simulink model "sg_xsvi_fanout"  (Simulink 7.6)
settings: Solver=ode45  StartTime=0.0  StopTime=1600.0  RelTol=1e-3
undefined symbols (not defined in the file): gcbh, xlBlockLoadCallback, xlGetNormalizedPeriod
libraries: xbsIndex_r4 x41, dspsrcs4 x6
settings Model: Creator=tbooth  LastModifiedBy=tawassne
settings OptimizationCC: InitFltsAndDblsToZero=on
settings DebuggingCC: SaveWithParameterizedLinksMsg=none  SignalResolutionControl=TryResolveAllWithWarning  MultiTaskDSMMsg=warning  MultiTaskCondExecSysMsg=none  StrictBusMsg=Warning
settings RTWCC: IncludeERTFirstTime=on
settings GRTTargetCC: TargetFcnLib=ansi_tfl_tmw.mat

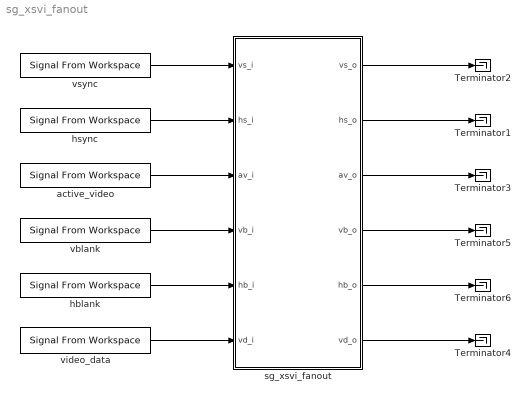
== system sg_xsvi_fanout ==
  Terminator{1..6} (6 alike) : Terminator
  active_video : dspsrcs4/Signal From Workspace  SystemSampleTime=-1  X="[ones(1,90) zeros(1,10)  ]"  Ts=1  nsamps=1  OutputAfterFinalValue=Cyclic repetition  ignoreOrWarnInputAndFrameLengths=off
  hblank : dspsrcs4/Signal From Workspace  SystemSampleTime=-1  X=[ zeros(1,1) ones(1,99) ]  Ts=1  nsamps=1  OutputAfterFinalValue=Cyclic repetition  ignoreOrWarnInputAndFrameLengths=off
  hsync : dspsrcs4/Signal From Workspace  SystemSampleTime=-1  X=[ zeros(1,1) ones(1,99) ]  Ts=1  nsamps=1  OutputAfterFinalValue=Cyclic repetition  ignoreOrWarnInputAndFrameLengths=off
  sg_xsvi_fanout : Subsystem
  vblank : dspsrcs4/Signal From Workspace  SystemSampleTime=-1  X=[ zeros(1,100) ones(1,900) ]  Ts=1  nsamps=1  OutputAfterFinalValue=Cyclic repetition  ignoreOrWarnInputAndFrameLengths=off
  video_data : dspsrcs4/Signal From Workspace  SystemSampleTime=-1  X=[repmat([10, 20],1,40),zeros(1,20), repmat([20,15],1,40) ,zeros(1,20)]  Ts=1  nsamps=1  OutputAfterFinalValue=Cyclic repetition  ignoreOrWarnInputAndFrameLengths=off
      link override From Workspace: OutputAfterFinalValue=Cyclic repetition
  vsync : dspsrcs4/Signal From Workspace  SystemSampleTime=-1  X=[ zeros(1,100) ones(1,900) ]  Ts=1  nsamps=1  OutputAfterFinalValue=Cyclic repetition  ignoreOrWarnInputAndFrameLengths=off
  wires:
  vsync/1 -> sg_xsvi_fanout/1(vs_i)
  hsync/1 -> sg_xsvi_fanout/2(hs_i)
  active_video/1 -> sg_xsvi_fanout/3(av_i)
  sg_xsvi_fanout/1(vs_o) -> Terminator2/1
  sg_xsvi_fanout/2(hs_o) -> Terminator1/1
  sg_xsvi_fanout/3(av_o) -> Terminator3/1
  sg_xsvi_fanout/6(vd_o) -> Terminator4/1
  video_data/1 -> sg_xsvi_fanout/6(vd_i)
  vblank/1 -> sg_xsvi_fanout/4(vb_i)
  hblank/1 -> sg_xsvi_fanout/5(hb_i)
  sg_xsvi_fanout/4(vb_o) -> Terminator5/1
  sg_xsvi_fanout/5(hb_o) -> Terminator6/1

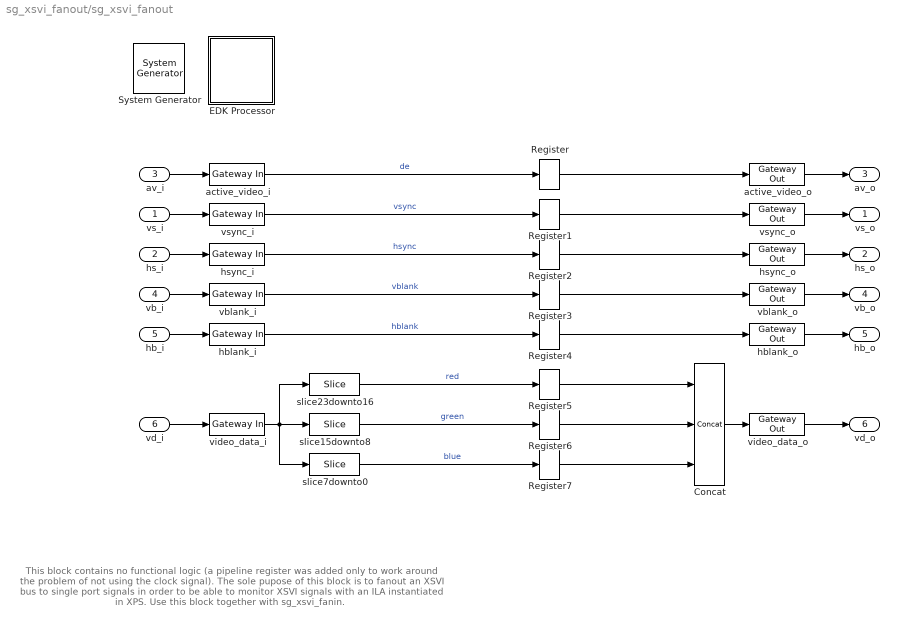
== system sg_xsvi_fanout/sg_xsvi_fanout ==
  note: This block contains no functional logic (a pipeline
      | register was added only to work around the problem
      | of not using the clock signal).
      | The sole pupose of this block is to fanout an XSVI bus
      | to single port signals in order to be able to monitor
      | XSVI signals with an ILA instantiated in XPS.
      |
      | Use this block together with sg_xsvi_fanin.
  vs_i : Inport
  hs_i : Inport  Port=2
  av_i : Inport  Port=3
  vb_i : Inport  Port=4
  hb_i : Inport  Port=5
  vd_i : Inport  Port=6
  " System Generator" : xbsIndex_r4/ System Generator  Tag=genX  SystemSampleTime=-1  xilinxfamily=spartan6  part=xc6slx150t  speed=-3  package=fgg676  synthesis_tool=XST  clock_wrapper=Clock Enables  directory=./export_edk  proj_type=Project Navigator  Synth_file=XST Defaults  Impl_file=ISE Defaults  testbench=off  simulink_period=1  sysclk_period=10  dcm_input_clock_period=10  incr_netlist=off  trim_vbits=Everywhere in SubSystem  dbl_ovrd=According to Block Masks  core_generation=According to Block Masks  run_coregen=off  deprecated_control=off  eval_field=0  block_type=sysgen
      settings: block_version=11.4
  Concat : xbsIndex_r4/Concat  num_inputs=3  dbl_ovrd=off  block_type=concat
  EDK Processor : Subsystem  LoadFcn=xlBlockLoadCallback(gcbh);  mask(Xilinx EDK Processor Block){mode=EDK pcore generation, xmp=, MemVisToProc=<qt bgcolor="#FFFFFF"></qt>, AvailableMemories=<empty>, portInterfaceTable={'exposed'=>[],'portdir'=>[],'portname'=>[],'shortname'=>[]}, bus_type_sgadvanced=, bus_type=PLB, baseaddr=0x80000000, baseaddr_lock_sgadvanced=, baseaddr_lock=off, dual_clock_sgadvanced=, dual_clock=on, reg_readback_sgadvanced=, reg_readback=on, ucf_file=, inheritDeviceType_sgadvanced=, inheritDeviceType=off, elf_file=, codebug_sgadvanced=, codebug=on, clock_name=plb, internalPortList={}, resetPolarity=0, memxtable={'mladdr'=>[],'mlist'=>[],'mlname'=>[],'mlstate'=>[]}, procinfo={}, memmapdirty=off, blockname=, xpsintstyle=default, has_advanced_control=0, sggui_pos=860,163,379,436, block_type=edkprocessor, block_version=2.7, sg_icon_stat=62,64,-1,-1,white,blue,0,07734,right,,[ ],[ ], sg_mask_display=|, sg_list_contents={'table'=>{'AvailableMemories'=>'popup(<empty>)'}}, sg_blockgui_xml=}
      mask sg_mask_display=|
      | fprintf('','COMMENT: begin icon graphics');
      | patch([0 62 62 0 0 ],[0 0 64 64 0 ],[0.77 0.82 0.91 ]);
      | plot([0 62 62 0 0 ],[0 0 64 64 0 ]);
      | patch([13.2 24.76 32.76 40.76 48.76 32.76 21.2 13.2 ],[40.88 40.88 48.88 40.88 48.88 48.88 48.88 40.88 ],[1 1 1 ]);
      | patch([21.2 32.76 24.76 13.2 21.2 ],[32.88 32.88 40.88 40.88 32.88 ],[0.931 0.946 0.973 ]);
      | patch([13.2 24.76 32.76 21.2 13.2 ],[24.88 24.88 32.88 32.88 24.88 ],[1 1 1 ]);
      | patch([21.2 48.76 40.76 32.76 24.76 13.2 21.2 ],[16.88 16.88 24.88 16.88 24.88 24.88 16.88 ],[0.931 0.946 0.973 ]);
      | fprintf('','COMMENT: end icon graphics');
      | fprintf('','COMMENT: begin icon text');
      | fprintf('','COMMENT: end icon text');
      mask prompts: mode "Configure Processor for"; xmp "XPS Project"; MemVisToProc ""; AvailableMemories "Available Memories"; portInterfaceTable ""; bus_type_sgadvanced ""; bus_type "Bus Type"; baseaddr "Base Address"; baseaddr_lock_sgadvanced ""; baseaddr_lock "Lock"; dual_clock_sgadvanced ""; dual_clock "Dual Clocks"; reg_readback_sgadvanced ""; reg_readback "Register Read-Back"; ucf_file "Constraint File"; inheritDeviceType_sgadvanced ""; inheritDeviceType "Inherit Device Type"; elf_file "Initial Program"; codebug_sgadvanced ""; codebug "Enable Co-Debug with Xilinx SDK (Beta)"; clock_name ""; internalPortList ""; resetPolarity ""; memxtable ""; procinfo ""; memmapdirty ""; blockname ""; xpsintstyle ""; has_advanced_control ""; sggui_pos ""; block_type ""; block_version ""; sg_icon_stat ""; sg_mask_display ""; sg_list_contents ""; sg_blockgui_xml ""
      mask help: Xilinx EDK Processor
      mask init:
      | try
      |   tmp_gcb = gcb;
      |   tmp_gcbh = gcbh;
      |   if (strcmp('SysGenIndex',get_param(bdroot(tmp_gcbh),'tag')) && ~isempty(regexp(bdroot(tmp_gcb), '^xbs', 'once')))
      |     return;
      |   end;
      |   xlMungeMaskParams;
      | 
      |   block_type='edkprocessor';
      | 
      |   serialized_declarations = '{''block_type''=>''String''}';
      |   xledkprocessor_init();
      |   ptable_ = xlblockprep(get_param(tmp_gcb, 'MaskWSVariables'));
      |   try
      |     xlBlockMoveCallback(tmp_gcbh);
      |   catch 
      |      clear global xl_updateicon_recursion_guard;
      |   end;
      | catch
      |   global dbgsysgen;
      |   if(~isempty(dbgsysgen) && dbgsysgen)
      |     e = regexprep(lasterr, '\n', '\nError: ');
      |     disp(['Error: While running MaskInit code on block ' tmp_gcb ': ' e]);
      |     error(e);
      |   end
      | end
      settings: CopyFcn=xlProcBlockCopyCallback(gcbh);xlBlockMoveCallback(gcbh);  DeleteFcn=xlDestroyGui(gcbh);  ModelCloseFcn=xlDestroyGui(gcbh);  PreSaveFcn=xlBlockPreSaveCallback(gcbh);  PostSaveFcn=xlBlockPostSaveCallback(gcbh);  DestroyFcn=xlDestroyGui(gcbh);  OpenFcn=bh=gcbh;xlProcBlockCallbacks('populatesharedmemorylistbox',bh);xlOpenGui(bh, 'edkprocessor_gui.xml', @xlProcBlockEnablement, @xlProcBlockAction);  CloseFcn=xlDestroyGui(gcbh);  MoveFcn=xlBlockMoveCallback(gcbh);
      mask Help: eval('');xlDoc('-book','sysgen','-topic','EDK_Processor');
      mask StyleString: popup(EDK pcore generation|HDL netlisting),edit,edit,edit,edit,edit,popup(AXI|PLB),edit,edit,checkbox,edit,checkbox,edit,checkbox,edit,edit,checkbox,edit,edit,checkbox,edit,edit,edit,edit,edit,edit,edit,edit,edit,edit,edit,edit,edit,edit,edit,edit
      mask Display:
      | fprintf('','COMMENT: begin icon graphics');
      | patch([0 62 62 0 0 ],[0 0 64 64 0 ],[0.77 0.82 0.91 ]);
      | plot([0 62 62 0 0 ],[0 0 64 64 0 ]);
      | patch([13.2 24.76 32.76 40.76 48.76 32.76 21.2 13.2 ],[40.88 40.88 48.88 40.88 48.88 48.88 48.88 40.88 ],[1 1 1 ]);
      | patch([21.2 32.76 24.76 13.2 21.2 ],[32.88 32.88 40.88 40.88 32.88 ],[0.931 0.946 0.973 ]);
      | patch([13.2 24.76 32.76 21.2 13.2 ],[24.88 24.88 32.88 32.88 24.88 ],[1 1 1 ]);
      | patch([21.2 48.76 40.76 32.76 24.76 13.2 21.2 ],[16.88 16.88 24.88 16.88 24.88 24.88 16.88 ],[0.931 0.946 0.973 ]);
      | fprintf('','COMMENT: end icon graphics');
      | fprintf('','COMMENT: begin icon text');
      | disp('');
      | 
      | fprintf('','COMMENT: end icon text');
  Register{,1..7} (8 alike) : xbsIndex_r4/Register  init=0  rst=off  en=off  dbl_ovrd=off  block_type=register
  active_video_i : xbsIndex_r4/Gateway In  gui_display_data_type=Fixed-point  arith_type=Unsigned  n_bits=1  bin_pt=0  preci_type=Single  exp_width=8  frac_width=24  quantization="Round  (unbiased: +/- Inf)"  overflow=Saturate  period=1  dbl_ovrd=off  timing_constraint=None  locs_specified=off  LOCs={}  hdl_port=on  block_type=gatewayin
      settings: infoedit="Gateway in block.  Converts inputs of type Simulink integer, double and fixed point to  Xilinx fixed point type.<P><P>Hardware notes:  In hardware these blocks become top level input ports."  xl_area=[0, 0, 0, 0, 0, 0, 0]  block_version=VER_STRING_GOES_HERE
  active_video_o : xbsIndex_r4/Gateway Out  hdl_port=on  timing_constraint=None  locs_specified=off  LOCs={}  block_type=gatewayout
      settings: infoedit="Gateway out block.  Converts Xilinx fixed point inputs into ouputs of type Simulink integer, double, or fixed point.<P><P>Hardware notes:  In hardware these blocks become top level output ports or are discarded, depending on how they are configured."  xl_area=[0, 0, 0, 0, 0, 0, 0]  block_version=VER_STRING_GOES_HERE
  hblank_i : xbsIndex_r4/Gateway In  gui_display_data_type=Fixed-point  arith_type=Unsigned  n_bits=1  bin_pt=0  preci_type=Single  exp_width=8  frac_width=24  quantization="Round  (unbiased: +/- Inf)"  overflow=Saturate  period=1  dbl_ovrd=off  timing_constraint=None  locs_specified=off  LOCs={}  hdl_port=on  block_type=gatewayin
      settings: infoedit="Gateway in block.  Converts inputs of type Simulink integer, double and fixed point to  Xilinx fixed point type.<P><P>Hardware notes:  In hardware these blocks become top level input ports."  xl_area=[0, 0, 0, 0, 0, 0, 0]  block_version=VER_STRING_GOES_HERE
  hblank_o : xbsIndex_r4/Gateway Out  hdl_port=on  timing_constraint=None  locs_specified=off  LOCs={}  block_type=gatewayout
      settings: infoedit="Gateway out block.  Converts Xilinx fixed point inputs into ouputs of type Simulink integer, double, or fixed point.<P><P>Hardware notes:  In hardware these blocks become top level output ports or are discarded, depending on how they are configured."  xl_area=[0, 0, 0, 0, 0, 0, 0]  block_version=VER_STRING_GOES_HERE
  hsync_i : xbsIndex_r4/Gateway In  gui_display_data_type=Fixed-point  arith_type=Unsigned  n_bits=1  bin_pt=0  preci_type=Single  exp_width=8  frac_width=24  quantization="Round  (unbiased: +/- Inf)"  overflow=Saturate  period=1  dbl_ovrd=off  timing_constraint=None  locs_specified=off  LOCs={}  hdl_port=on  block_type=gatewayin
      settings: infoedit="Gateway in block.  Converts inputs of type Simulink integer, double and fixed point to  Xilinx fixed point type.<P><P>Hardware notes:  In hardware these blocks become top level input ports."  xl_area=[0, 0, 0, 0, 0, 0, 0]  block_version=VER_STRING_GOES_HERE
  hsync_o : xbsIndex_r4/Gateway Out  hdl_port=on  timing_constraint=None  locs_specified=off  LOCs={}  block_type=gatewayout
      settings: infoedit="Gateway out block.  Converts Xilinx fixed point inputs into ouputs of type Simulink integer, double, or fixed point.<P><P>Hardware notes:  In hardware these blocks become top level output ports or are discarded, depending on how they are configured."  xl_area=[0, 0, 0, 0, 0, 0, 0]  block_version=VER_STRING_GOES_HERE
  slice15downto8 : xbsIndex_r4/Slice  nbits=8  boolean_output=off  mode=Lower Bit Location + Width  bit1=0  base1=MSB of Input  bit0=8  base0=LSB of Input  dbl_ovrd=off  block_type=slice
  slice23downto16 : xbsIndex_r4/Slice  nbits=8  boolean_output=off  mode=Lower Bit Location + Width  bit1=0  base1=MSB of Input  bit0=16  base0=LSB of Input  dbl_ovrd=off  block_type=slice
  slice7downto0 : xbsIndex_r4/Slice  nbits=8  boolean_output=off  mode=Lower Bit Location + Width  bit1=0  base1=MSB of Input  bit0=0  base0=LSB of Input  dbl_ovrd=off  block_type=slice
  vblank_i : xbsIndex_r4/Gateway In  gui_display_data_type=Fixed-point  arith_type=Unsigned  n_bits=1  bin_pt=0  preci_type=Single  exp_width=8  frac_width=24  quantization="Round  (unbiased: +/- Inf)"  overflow=Saturate  period=1  dbl_ovrd=off  timing_constraint=None  locs_specified=off  LOCs={}  hdl_port=on  block_type=gatewayin
      settings: infoedit="Gateway in block.  Converts inputs of type Simulink integer, double and fixed point to  Xilinx fixed point type.<P><P>Hardware notes:  In hardware these blocks become top level input ports."  xl_area=[0, 0, 0, 0, 0, 0, 0]  block_version=VER_STRING_GOES_HERE
  vblank_o : xbsIndex_r4/Gateway Out  hdl_port=on  timing_constraint=None  locs_specified=off  LOCs={}  block_type=gatewayout
      settings: infoedit="Gateway out block.  Converts Xilinx fixed point inputs into ouputs of type Simulink integer, double, or fixed point.<P><P>Hardware notes:  In hardware these blocks become top level output ports or are discarded, depending on how they are configured."  xl_area=[0, 0, 0, 0, 0, 0, 0]  block_version=VER_STRING_GOES_HERE
  video_data_i : xbsIndex_r4/Gateway In  gui_display_data_type=Fixed-point  arith_type=Unsigned  n_bits=24  bin_pt=0  preci_type=Single  exp_width=8  frac_width=24  quantization="Round  (unbiased: +/- Inf)"  overflow=Saturate  period=1  dbl_ovrd=off  timing_constraint=None  locs_specified=off  LOCs={}  hdl_port=on  block_type=gatewayin
      settings: infoedit="Gateway in block.  Converts inputs of type Simulink integer, double and fixed point to  Xilinx fixed point type.<br><br>Hardware notes:  In hardware these blocks become top level input ports."  xl_area=[0, 0, 0, 0, 0, 0, 0]  block_version=VER_STRING_GOES_HERE
  video_data_o : xbsIndex_r4/Gateway Out  hdl_port=on  timing_constraint=None  locs_specified=off  LOCs={}  block_type=gatewayout
      settings: infoedit="Gateway out block.  Converts Xilinx fixed point inputs into ouputs of type Simulink integer, double, or fixed point.<P><P>Hardware notes:  In hardware these blocks become top level output ports or are discarded, depending on how they are configured."  xl_area=[0, 0, 0, 0, 0, 0, 0]  block_version=VER_STRING_GOES_HERE
  vsync_i : xbsIndex_r4/Gateway In  gui_display_data_type=Fixed-point  arith_type=Unsigned  n_bits=1  bin_pt=0  preci_type=Single  exp_width=8  frac_width=24  quantization="Round  (unbiased: +/- Inf)"  overflow=Saturate  period=1  dbl_ovrd=off  timing_constraint=None  locs_specified=off  LOCs={}  hdl_port=on  block_type=gatewayin
      settings: infoedit="Gateway in block.  Converts inputs of type Simulink integer, double and fixed point to  Xilinx fixed point type.<P><P>Hardware notes:  In hardware these blocks become top level input ports."  xl_area=[0, 0, 0, 0, 0, 0, 0]  block_version=VER_STRING_GOES_HERE
  vsync_o : xbsIndex_r4/Gateway Out  hdl_port=on  timing_constraint=None  locs_specified=off  LOCs={}  block_type=gatewayout
      settings: infoedit="Gateway out block.  Converts Xilinx fixed point inputs into ouputs of type Simulink integer, double, or fixed point.<P><P>Hardware notes:  In hardware these blocks become top level output ports or are discarded, depending on how they are configured."  xl_area=[0, 0, 0, 0, 0, 0, 0]  block_version=VER_STRING_GOES_HERE
  vs_o : Outport
  hs_o : Outport  Port=2
  av_o : Outport  Port=3
  vb_o : Outport  Port=4
  hb_o : Outport  Port=5
  vd_o : Outport  Port=6
  wires:
  active_video_i/1 -> Register/1  "de"
  vsync_i/1 -> Register1/1  "vsync"
  av_i/1 -> active_video_i/1
  vs_i/1 -> vsync_i/1
  hs_i/1 -> hsync_i/1
  vd_i/1 -> video_data_i/1
  active_video_o/1 -> av_o/1
  vsync_o/1 -> vs_o/1
  hsync_o/1 -> hs_o/1
  Concat/1 -> video_data_o/1
  slice23downto16/1 -> Register5/1  "red"
  slice15downto8/1 -> Register6/1  "green"
  vblank_o/1 -> vb_o/1
  hblank_o/1 -> hb_o/1
  vb_i/1 -> vblank_i/1
  hb_i/1 -> hblank_i/1
  vblank_i/1 -> Register3/1  "vblank"
  hblank_i/1 -> Register4/1  "hblank"
  video_data_i/1 -> slice15downto8/1, slice23downto16/1, slice7downto0/1
  hsync_i/1 -> Register2/1  "hsync"
  slice7downto0/1 -> Register7/1  "blue"
  video_data_o/1 -> vd_o/1
  Register/1 -> active_video_o/1
  Register1/1 -> vsync_o/1
  Register2/1 -> hsync_o/1
  Register3/1 -> vblank_o/1
  Register4/1 -> hblank_o/1
  Register5/1 -> Concat/1
  Register6/1 -> Concat/2
  Register7/1 -> Concat/3

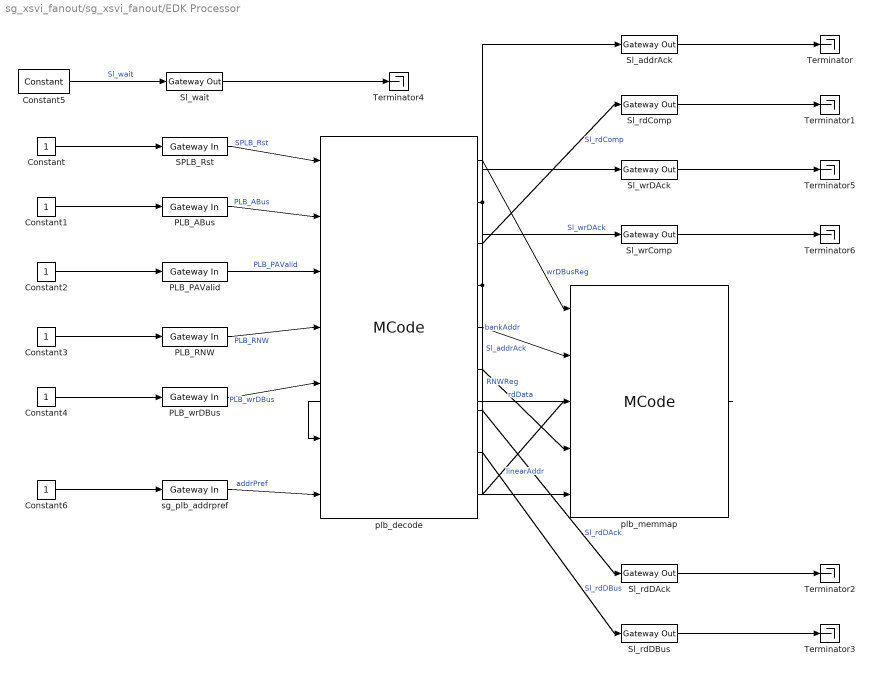
== system sg_xsvi_fanout/sg_xsvi_fanout/EDK Processor ==
  Constant{,1..4,6} (6 alike) : Constant
  Constant5 : xbsIndex_r4/Constant  const=0  gui_display_data_type=Fixed-point  arith_type=Unsigned  n_bits=1  bin_pt=0  preci_type=Single  exp_width=8  frac_width=24  explicit_period=on  period=xlGetNormalizedPeriod()  equ=P=C  opselect=C  inp2=PCIN>>17  opr=+  inp1=P  carry=CIN  dbl_ovrd=off  block_type=constant
  PLB_ABus : xbsIndex_r4/Gateway In  gui_display_data_type=Fixed-point  arith_type=Unsigned  n_bits=32  bin_pt=0  preci_type=Single  exp_width=8  frac_width=24  quantization="Round  (unbiased: +/- Inf)"  overflow=Saturate  period=xlGetNormalizedPeriod()  dbl_ovrd=off  timing_constraint=None  locs_specified=off  LOCs={}  hdl_port=on  block_type=gatewayin
      settings: infoedit="Gateway in block.  Converts inputs of type Simulink integer, double and fixed point to  Xilinx fixed point or floating-point data type.<br><br>Hardware notes:  In hardware these blocks become top level input ports."  sginterface={'Xilinx'=>{'jtaghwcosim'=>{'non_memory_mapped_port'=>'PLB_ABus'}},'iopad'=>{'constraint'=>'#'}}
  PLB_PAValid : xbsIndex_r4/Gateway In  gui_display_data_type=Fixed-point  arith_type=Unsigned  n_bits=1  bin_pt=0  preci_type=Single  exp_width=8  frac_width=24  quantization="Round  (unbiased: +/- Inf)"  overflow=Saturate  period=xlGetNormalizedPeriod()  dbl_ovrd=off  timing_constraint=None  locs_specified=off  LOCs={}  hdl_port=on  block_type=gatewayin
      settings: infoedit="Gateway in block.  Converts inputs of type Simulink integer, double and fixed point to  Xilinx fixed point or floating-point data type.<br><br>Hardware notes:  In hardware these blocks become top level input ports."  sginterface={'Xilinx'=>{'jtaghwcosim'=>{'non_memory_mapped_port'=>'PLB_PAValid'}},'iopad'=>{'constraint'=>'#'}}
  PLB_RNW : xbsIndex_r4/Gateway In  gui_display_data_type=Fixed-point  arith_type=Unsigned  n_bits=1  bin_pt=0  preci_type=Single  exp_width=8  frac_width=24  quantization="Round  (unbiased: +/- Inf)"  overflow=Saturate  period=xlGetNormalizedPeriod()  dbl_ovrd=off  timing_constraint=None  locs_specified=off  LOCs={}  hdl_port=on  block_type=gatewayin
      settings: infoedit="Gateway in block.  Converts inputs of type Simulink integer, double and fixed point to  Xilinx fixed point or floating-point data type.<br><br>Hardware notes:  In hardware these blocks become top level input ports."  sginterface={'Xilinx'=>{'jtaghwcosim'=>{'non_memory_mapped_port'=>'PLB_RNW'}},'iopad'=>{'constraint'=>'#'}}
  PLB_wrDBus : xbsIndex_r4/Gateway In  gui_display_data_type=Fixed-point  arith_type=Unsigned  n_bits=32  bin_pt=0  preci_type=Single  exp_width=8  frac_width=24  quantization="Round  (unbiased: +/- Inf)"  overflow=Saturate  period=xlGetNormalizedPeriod()  dbl_ovrd=off  timing_constraint=None  locs_specified=off  LOCs={}  hdl_port=on  block_type=gatewayin
      settings: infoedit="Gateway in block.  Converts inputs of type Simulink integer, double and fixed point to  Xilinx fixed point or floating-point data type.<br><br>Hardware notes:  In hardware these blocks become top level input ports."  sginterface={'Xilinx'=>{'jtaghwcosim'=>{'non_memory_mapped_port'=>'PLB_wrDBus'}},'iopad'=>{'constraint'=>'#'}}
  SPLB_Rst : xbsIndex_r4/Gateway In  gui_display_data_type=Fixed-point  arith_type=Unsigned  n_bits=1  bin_pt=0  preci_type=Single  exp_width=8  frac_width=24  quantization="Round  (unbiased: +/- Inf)"  overflow=Saturate  period=xlGetNormalizedPeriod()  dbl_ovrd=off  timing_constraint=None  locs_specified=off  LOCs={}  hdl_port=on  block_type=gatewayin
      settings: infoedit="Gateway in block.  Converts inputs of type Simulink integer, double and fixed point to  Xilinx fixed point or floating-point data type.<br><br>Hardware notes:  In hardware these blocks become top level input ports."  sginterface={'Xilinx'=>{'jtaghwcosim'=>{'non_memory_mapped_port'=>'SPLB_Rst'}},'iopad'=>{'constraint'=>'#'}}
  Sl_addrAck : xbsIndex_r4/Gateway Out  hdl_port=on  timing_constraint=None  locs_specified=off  LOCs={}  block_type=gatewayout
      settings: infoedit="Gateway out block.  Converts Xilinx fixed point or floating-point type inputs into ouputs of type Simulink integer, double, or fixed point.<br><br>Hardware notes:  In hardware these blocks become top level output ports or are discarded, depending on how they are configured."  sginterface={'Xilinx'=>{'jtaghwcosim'=>{'non_memory_mapped_port'=>'Sl_addrAck'}},'iopad'=>{'constraint'=>'#'}}
  Sl_rdComp : xbsIndex_r4/Gateway Out  hdl_port=on  timing_constraint=None  locs_specified=off  LOCs={}  block_type=gatewayout
      settings: infoedit="Gateway out block.  Converts Xilinx fixed point or floating-point type inputs into ouputs of type Simulink integer, double, or fixed point.<br><br>Hardware notes:  In hardware these blocks become top level output ports or are discarded, depending on how they are configured."  sginterface={'Xilinx'=>{'jtaghwcosim'=>{'non_memory_mapped_port'=>'Sl_rdComp'}},'iopad'=>{'constraint'=>'#'}}
  Sl_rdDAck : xbsIndex_r4/Gateway Out  hdl_port=on  timing_constraint=None  locs_specified=off  LOCs={}  block_type=gatewayout
      settings: infoedit="Gateway out block.  Converts Xilinx fixed point or floating-point type inputs into ouputs of type Simulink integer, double, or fixed point.<br><br>Hardware notes:  In hardware these blocks become top level output ports or are discarded, depending on how they are configured."  sginterface={'Xilinx'=>{'jtaghwcosim'=>{'non_memory_mapped_port'=>'Sl_rdDAck'}},'iopad'=>{'constraint'=>'#'}}
  Sl_rdDBus : xbsIndex_r4/Gateway Out  hdl_port=on  timing_constraint=None  locs_specified=off  LOCs={}  block_type=gatewayout
      settings: infoedit="Gateway out block.  Converts Xilinx fixed point or floating-point type inputs into ouputs of type Simulink integer, double, or fixed point.<br><br>Hardware notes:  In hardware these blocks become top level output ports or are discarded, depending on how they are configured."  sginterface={'Xilinx'=>{'jtaghwcosim'=>{'non_memory_mapped_port'=>'Sl_rdDBus'}},'iopad'=>{'constraint'=>'#'}}
  Sl_wait : xbsIndex_r4/Gateway Out  hdl_port=on  timing_constraint=None  locs_specified=off  LOCs={}  block_type=gatewayout
      settings: infoedit="Gateway out block.  Converts Xilinx fixed point or floating-point type inputs into ouputs of type Simulink integer, double, or fixed point.<br><br>Hardware notes:  In hardware these blocks become top level output ports or are discarded, depending on how they are configured."  sginterface={'Xilinx'=>{'jtaghwcosim'=>{'non_memory_mapped_port'=>'Sl_wait'}},'iopad'=>{'constraint'=>'#'}}
  Sl_wrComp : xbsIndex_r4/Gateway Out  hdl_port=on  timing_constraint=None  locs_specified=off  LOCs={}  block_type=gatewayout
      settings: infoedit="Gateway out block.  Converts Xilinx fixed point or floating-point type inputs into ouputs of type Simulink integer, double, or fixed point.<br><br>Hardware notes:  In hardware these blocks become top level output ports or are discarded, depending on how they are configured."  sginterface={'Xilinx'=>{'jtaghwcosim'=>{'non_memory_mapped_port'=>'Sl_wrComp'}},'iopad'=>{'constraint'=>'#'}}
  Sl_wrDAck : xbsIndex_r4/Gateway Out  hdl_port=on  timing_constraint=None  locs_specified=off  LOCs={}  block_type=gatewayout
      settings: infoedit="Gateway out block.  Converts Xilinx fixed point or floating-point type inputs into ouputs of type Simulink integer, double, or fixed point.<br><br>Hardware notes:  In hardware these blocks become top level output ports or are discarded, depending on how they are configured."  sginterface={'Xilinx'=>{'jtaghwcosim'=>{'non_memory_mapped_port'=>'Sl_wrDAck'}},'iopad'=>{'constraint'=>'#'}}
  Terminator{,1..6} (7 alike) : Terminator
  plb_decode : xbsIndex_r4/MCode  mfname=xlmax  explicit_period=off  period=1  dbl_ovrd=off  enable_stdout=off  enable_debug=off  mfilecontent=|  suppress_output=on  defparams={}  hide_port_list={}  block_type=mcode
      | function [wrDBusReg, addrAck, rdComp, wrDAck, bankAddr, RNWReg, rdDAck, rdDBus, linearAddr] = plb_bus_decode(plbRst, plbABus, plbPAValid, plbRNW, plbWrDBus, rdData, addrPref)
      | 
      | % constant variables (TODO: should pass from outside)
      | ADDRPREF_LEN = 20;
      | BANKADDR_LEN = 2;
      | LINEARADDR_LEN = 8;
      | ABUS_LEN = 32;
      | DBUS_LEN = 32;
      | 
      | % declare and initialize persistent variables
      | % register input bus signals
      | persistent plbRstReg_, plbRstReg_ = xl_state(0, {xlBoolean});
      | persistent plbABusReg_, plbABusReg_ = xl_state(0, {xlUnsigned, ABUS_LEN, 0});
      | persistent plbPAValidReg_, plbPAValidReg_ = xl_state(0, {xlBoolean});
      | persistent plbRNWReg_, plbRNWReg_ = xl_state(0, {xlUnsigned, 1, 0});
      | persistent plbWrDBusReg_, plbWrDBusReg_ = xl_state(0, {xlUnsigned, DBUS_LEN, 0});
      | 
      | % ===== rest of the outputs =====
      | 
      | bankAddr   = xl_slice(plbABusReg_, 2+BANKADDR_LEN+LINEARADDR_LEN-1, 2+LINEARADDR_LEN);
      | linearAddr = xl_slice(plbABusReg_, 2+LINEARADDR_LEN-1, 2);
      | RNWReg = plbRNWReg_;
      | wrDBusReg = plbWrDBusReg_;
      | 
      | % ===== p_select =====
      | 
      | % register PAValid
      | persistent aValidReg, aValidReg = xl_state(0, {xlBoolean});
      | aValidReg = plbPAValidReg_;
      | 
      | % extract and register the address prefix
      | addrPref_in = xl_slice(plbABusReg_, xl_nbits(plbABusReg_)-1, xl_nbits(plbABusReg_)-ADDRPREF_LEN);
      | if addrPref_in == addrPref
      |     ps1 = true;
      | else 
      |     ps1 = false;
      | end 
      | 
      | persistent ps1Reg, ps1Reg = xl_state(0, ps1);
      | ps1Reg = ps1;
      | 
      | ps = xl_and(ps1Reg, aValidReg);
      | 
      | % ===== addrAck =====
      | 
      | % register ps
      | persistent psReg, psReg = xl_state(0, ps);
      | 
      | addrAck = xfix({xlUnsigned, 1, 0}, xl_and(xl_not(plbRstReg_), ps, xl_not(psReg)));
      | 
      | psReg = ps;
      | 
      | % ===== rdComp, rd/wr DAck =====
      |  
      | rdComp1 = xfix({xlUnsigned, 1, 0}, xl_and(addrAck, RNWReg));
      | 
      | NUM_rdCompDelay = 3;
      | persistent rdCompDelay, rdCompDelay = xl_state(zeros(1, NUM_rdCompDelay), rdComp1, NUM_rdCompDelay);
      | rdComp2 = rdCompDelay.back;
      | rdCompDelay.push_front_pop_back(rdComp1);
      | 
      | persistent rdCompReg, rdCompReg = xl_state(0, rdComp1);
      | rdComp = rdCompReg;
      | rdCompReg = rdComp2;
      | 
      | persistent rdDAckReg, rdDAckReg = xl_state(0, rdComp1);
      | rdDAck = rdDAckReg;
      | rdDAckReg = rdComp;
      | 
      | persistent wrDAckReg, wrDAckReg = xl_state(0, addrAck);
      | wrDAck = wrDAckReg;
      | wrDAckReg = xl_and(addrAck, xl_not(RNWReg));
      | 
      | % ===== rdDBus =====
      | 
      | rdSel = xl_or(rdComp2, rdComp);
      | 
      | if rdSel == 1
      |     rdDBus1 = rdData;
      | else
      |     rdDBus1 = 0;
      | end % if
      | 
      | persistent rdDBusReg, rdDBusReg = xl_state(0, rdDBus1);
      | rdDBus = rdDBusReg;
      | rdDBusReg = rdDBus1;
      | 
      | % rdDBus = xl_concat(rdDBus32, rdDBus32);
      | % rdDBus = rdDBus32;
      | 
      | % ===== update the persistent variables =====
      | 
      | plbRstReg_ = plbRst;
      | plbABusReg_ = plbABus;
      | plbPAValidReg_ = plbPAValid;
      | plbRNWReg_ = plbRNW;
      | plbWrDBusReg_ = xl_slice(plbWrDBus, DBUS_LEN-1, 0);
  plb_memmap : xbsIndex_r4/MCode  mfname=xlmax  explicit_period=off  period=1  dbl_ovrd=off  enable_stdout=off  enable_debug=off  mfilecontent=|  suppress_output=on  defparams={}  hide_port_list={}  block_type=mcode
      | function [read_bank_out] = plb_memmap(wrDBus, bankAddr, linearAddr, RNWReg, addrAck)
      | 
      | 
      | % connvert the input data to UFix_32_0 (the bus data type)
      | % 'From Register' blocks
      | % 'To Register' blocks
      | 
      | % 'From FIFO' blocks
      | % 'To FIFO' blocks
      | % 'Shared Memory' blocks
      | 
      | % 'dout' ports of 'From Register' blocks
      | 
      | 
      | % 'From FIFO' and 'To FIFO' blocks
      | 
      | 
      | 
      | 
      | 
      | opCode = xl_concat(addrAck, RNWReg, bankAddr, linearAddr);
      | 
      | % 'Shared Memory' blocks
      | 
      | 
      | 
      | 
      | 
      | % 'din' ports of 'Shared Memory' blocks
      | 
      | 
      | % 'we' ports of 'Shared Memory' blocks
      | 
      | 
      | % 'addr' ports of 'Shared Memory' blocks
      | 
      | 
      | % 're' ports of 'From FIFO' blocks
      | 
      | 
      | % 'en' ports of 'To Register' blocks
      | 
      | 
      | % 'din' ports of 'To FIFO' blocks
      | 
      | 
      | % 'we' ports of 'To FIFO' blocks
      | 
      | 
      | % 'din' ports of 'To Register' blocks
      | 
      | 
      | persistent read_bank_out_reg; read_bank_out_reg = xl_state(0, {xlUnsigned, 32, 0});
      | read_bank_out = read_bank_out_reg;
      | 
      | persistent bankAddr_reg; bankAddr_reg = xl_state(0, bankAddr);
      | 
      | if bankAddr_reg == 0
      |     % Bank 0: Shared Memories
      |     read_bank_out_reg = 0;
      | elseif bankAddr_reg == 1
      |     % Bank 1: From/To FIFOs
      |     read_bank_out_reg =  0;
      | elseif bankAddr_reg == 2
      |     % Bank 2: From/To Registers
      |     read_bank_out_reg = 0;
      | elseif bankAddr_reg == 3
      |     % Bank 3: Configuration Registers
      |     read_bank_out_reg = 0;
      | end
      | 
      | bankAddr_reg = bankAddr;
  sg_plb_addrpref : xbsIndex_r4/Gateway In  gui_display_data_type=Fixed-point  arith_type=Unsigned  n_bits=20  bin_pt=0  preci_type=Single  exp_width=8  frac_width=24  quantization="Round  (unbiased: +/- Inf)"  overflow=Saturate  period=xlGetNormalizedPeriod()  dbl_ovrd=off  timing_constraint=None  locs_specified=off  LOCs={}  hdl_port=on  block_type=gatewayin
      settings: infoedit="Gateway in block.  Converts inputs of type Simulink integer, double and fixed point to  Xilinx fixed point or floating-point data type.<br><br>Hardware notes:  In hardware these blocks become top level input ports."  sginterface={'Xilinx'=>{'jtaghwcosim'=>{'non_memory_mapped_port'=>'sg_plb_addrpref'}},'iopad'=>{'constraint'=>'#'}}
  wires:
  plb_decode/2 -> plb_memmap/5, Sl_addrAck/1  "Sl_addrAck"
  plb_decode/4 -> Sl_wrDAck/1, Sl_wrComp/1  "Sl_wrDAck"
  plb_memmap/1 -> plb_decode/6  "rdData"
  plb_decode/6 -> plb_memmap/4  "RNWReg"
  plb_decode/9 -> plb_memmap/3  "linearAddr"
  plb_decode/5 -> plb_memmap/2  "bankAddr"
  plb_decode/1 -> plb_memmap/1  "wrDBusReg"
  plb_decode/8 -> Sl_rdDBus/1  "Sl_rdDBus"
  plb_decode/7 -> Sl_rdDAck/1  "Sl_rdDAck"
  plb_decode/3 -> Sl_rdComp/1  "Sl_rdComp"
  sg_plb_addrpref/1 -> plb_decode/7  "addrPref"
  PLB_wrDBus/1 -> plb_decode/5  "PLB_wrDBus"
  PLB_RNW/1 -> plb_decode/4  "PLB_RNW"
  PLB_PAValid/1 -> plb_decode/3  "PLB_PAValid"
  PLB_ABus/1 -> plb_decode/2  "PLB_ABus"
  SPLB_Rst/1 -> plb_decode/1  "SPLB_Rst"
  Constant6/1 -> sg_plb_addrpref/1
  Constant5/1 -> Sl_wait/1  "Sl_wait"
  Constant4/1 -> PLB_wrDBus/1
  Constant3/1 -> PLB_RNW/1
  Constant2/1 -> PLB_PAValid/1
  Constant1/1 -> PLB_ABus/1
  Constant/1 -> SPLB_Rst/1
  Sl_wrComp/1 -> Terminator6/1
  Sl_wrDAck/1 -> Terminator5/1
  Sl_wait/1 -> Terminator4/1
  Sl_rdDBus/1 -> Terminator3/1
  Sl_rdDAck/1 -> Terminator2/1
  Sl_rdComp/1 -> Terminator1/1
  Sl_addrAck/1 -> Terminator/1
